simulink library "AdvancedDemux"  (R2014b)
settings: Solver=ode45  StartTime=0.0  StopTime=10.0  RelTol=1e-3
settings Model: Creator=Hp  LastModifiedBy=Hp

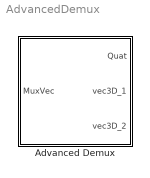
== system AdvancedDemux ==
  Advanced Demux : Subsystem

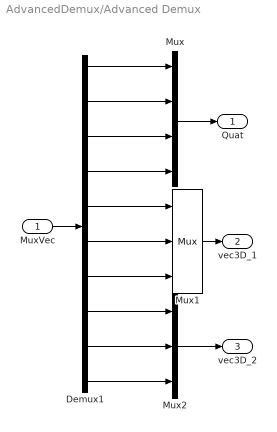
== system AdvancedDemux/Advanced Demux ==
  MuxVec : Inport
  Demux1 : Demux  Outputs=10
  Mux : Mux
  Mux1 : Mux  Inputs=3
  Mux2 : Mux  Inputs=3
  Quat : Outport
  vec3D_1 : Outport  Port=2
  vec3D_2 : Outport  Port=3
  wires:
  Demux1/7 -> Mux1/3
  Demux1/9 -> Mux2/2
  Demux1/6 -> Mux1/2
  Mux1/1 -> vec3D_1/1
  MuxVec/1 -> Demux1/1
  Mux/1 -> Quat/1
  Mux2/1 -> vec3D_2/1
  Demux1/2 -> Mux/2
  Demux1/1 -> Mux/1
  Demux1/8 -> Mux2/1
  Demux1/4 -> Mux/4
  Demux1/3 -> Mux/3
  Demux1/10 -> Mux2/3
  Demux1/5 -> Mux1/1
